simulink model "simulink_controlTemperatura"  (R2022b)
settings: Solver=VariableStepAuto  StartTime=0.0  StopTime=10.0  RelTol=1e-3
libraries: fuzblock x1
settings Model: Creator=KeOnd  LastModifiedBy=KeOnd

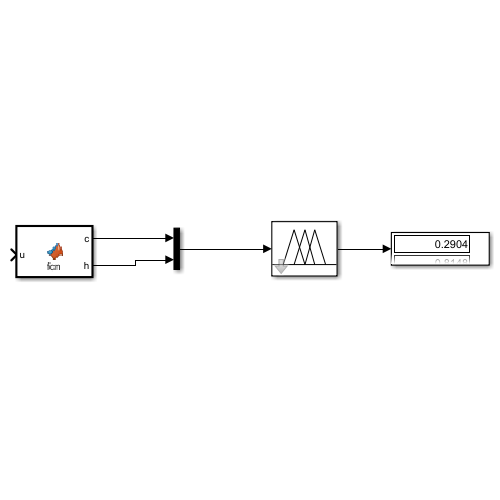
[thumbnail: Simulink's stored preview of the top-level diagram]
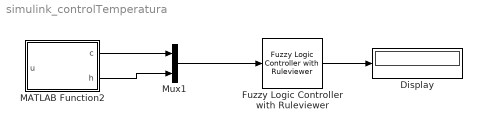
== system simulink_controlTemperatura ==
  Display : Display
  Fuzzy Logic Controller with Ruleviewer : fuzblock/Fuzzy Logic  Controller  with Ruleviewer  fismatrix=temp4  Ts=2
  MATLAB Function2 : MATLAB Function  TreatAsAtomicUnit=on
  Mux1 : Mux  Inputs=2
  wires:
  Fuzzy Logic Controller with Ruleviewer/1 -> Display/1
  Mux1/1 -> Fuzzy Logic Controller with Ruleviewer/1
  MATLAB Function2/1(c) -> Mux1/1
  MATLAB Function2/2(h) -> Mux1/2

== matlab function simulink_controlTemperatura/MATLAB Function2 ==
  data: u input; c output; h output
function [c, h] = fcn(u)

coder.extrinsic('pyrunfile')
temperatura = zeros(size(u), 'double');
humidity = zeros(size(u), 'double');

temperatura = pyrunfile("weatherApi.py","celsius");
humidity = pyrunfile("weatherApi.py","humidity");

c = temperatura;
h = humidity;
